simulink model "power_conversion_system"  (R2026a)
settings: Solver=VariableStepAuto  StopTime=100e-3  MaxStep=10e-6  MinStep=1e-9
values from neighbouring files (symbols this model uses):
  C_out1 = 100e-6    (= 0.0001)    [power_system_variables.m]
  L_boost1 = 1e-3    (= 0.001)    [power_system_variables.m]
  R_Load = 10    [power_system_variables.m]
  R_sense1 = 0.1    [power_system_variables.m]
  Vin = 12    [power_system_variables.m]
  Vout = 48    [power_system_variables.m]
undefined symbols (not defined in the file or in its folder): f_clk
settings Model: Creator=codykremer  LastModifiedBy=codykremer

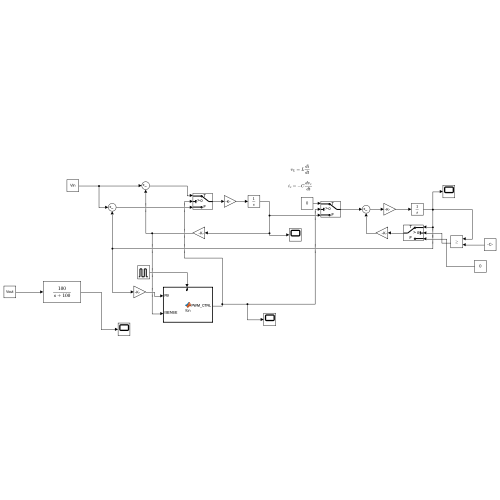
[thumbnail: Simulink's stored preview of the top-level diagram]
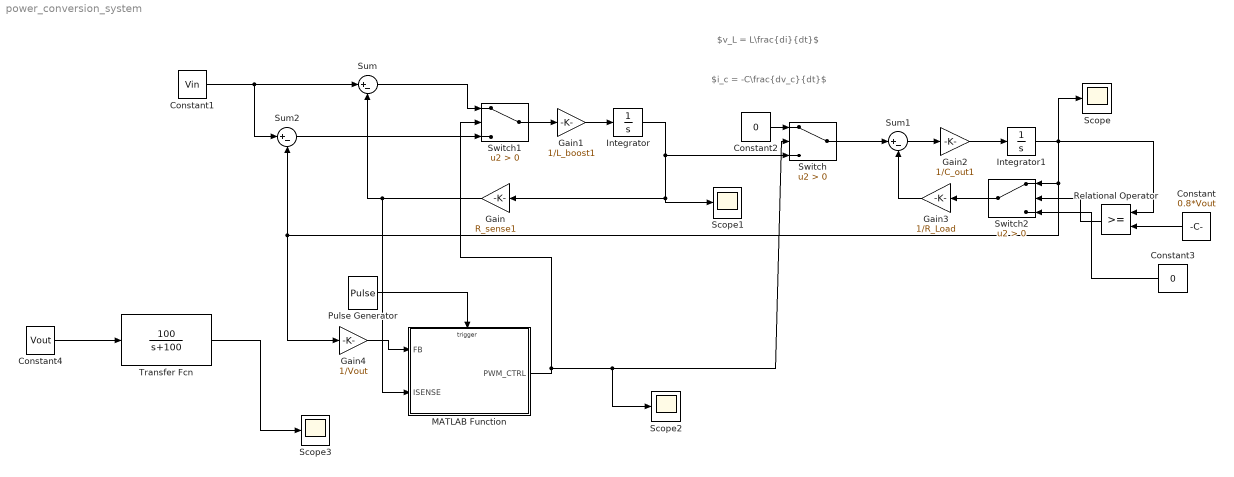
== system power_conversion_system ==
  note: $v_L = L\frac{di}{dt}$
  note: $i_c = -C\frac{dv_c}{dt}$
  Constant : Constant  Value=0.8*Vout  VectorParams1D=off
  Constant1 : Constant  Value=Vin
  Constant2 : Constant  Value=0
  Constant3 : Constant  Value=0  VectorParams1D=off
  Constant4 : Constant  Value=Vout
  Gain : Gain  Gain=R_sense1
  Gain1 : Gain  Gain=1/L_boost1
  Gain2 : Gain  Gain=1/C_out1
  Gain3 : Gain  Gain=1/R_Load
  Gain4 : Gain  Gain=1/Vout
  Integrator : Integrator
  Integrator1 : Integrator
  MATLAB Function : MATLAB Function  TreatAsAtomicUnit=on
  Pulse Generator : DiscretePulseGenerator  PulseType=Time based  Period=1/f_clk  PulseWidth=50
  Relational Operator : RelationalOperator  OutDataTypeStr=boolean  RndMeth=Simplest  InputSameDT=off
  Scope{,1..3} (4 alike) : Scope
      Scope settings: ActiveDisplayYMinimum=-3.0238183140973316  ActiveDisplayYMaximum=27.214364826875993
      Scope1 settings: ActiveDisplayYMinimum=-76.4299194528486  ActiveDisplayYMaximum=74.60389998830459
      Scope2 settings: ActiveDisplayYMinimum=-1  ActiveDisplayYMaximum=1  DataLoggingVariableName=ScopeData2
      Scope3 settings: ActiveDisplayYMinimum=-1  ActiveDisplayYMaximum=1  DataLoggingVariableName=ScopeData3
  Sum : Sum  Inputs=|+-
  Sum1 : Sum  Inputs=|+-
  Sum2 : Sum  Inputs=|+-
  Switch : Switch  Criteria=u2 > Threshold  SaturateOnIntegerOverflow=off  InputSameDT=off
  Switch1 : Switch  Criteria=u2 > Threshold  SaturateOnIntegerOverflow=off  InputSameDT=off
  Switch2 : Switch  Criteria=u2 > Threshold  SaturateOnIntegerOverflow=off  InputSameDT=off
  Transfer Fcn : TransferFcn  Numerator=[100]  Denominator=[1 100]
  wires:
  Sum1/1 -> Gain2/1
  Gain2/1 -> Integrator1/1
  Switch/1 -> Sum1/1
  Constant2/1 -> Switch/1
  Gain3/1 -> Sum1/2
  Constant1/1 -> Sum/1, Sum2/1
  Gain1/1 -> Integrator/1
  Sum/1 -> Switch1/1
  Integrator/1 -> Switch/3, Scope1/1, Gain/1
  Gain/1 -> Sum/2, MATLAB Function/2(ISENSE)
  Sum2/1 -> Switch1/3
  Switch1/1 -> Gain1/1
  Pulse Generator/1 -> MATLAB Function/Trigger
  MATLAB Function/1(PWM_CTRL) -> Scope2/1, Switch/2, Switch1/2
  Switch2/1 -> Gain3/1
  Constant/1 -> Relational Operator/2
  Relational Operator/1 -> Switch2/2
  Constant3/1 -> Switch2/3
  Integrator1/1 -> Relational Operator/1, Scope/1, Switch2/1, Gain4/1, Sum2/2
  Constant4/1 -> Transfer Fcn/1
  Gain4/1 -> MATLAB Function/1(FB)
  Transfer Fcn/1 -> Scope3/1

== matlab function power_conversion_system/MATLAB Function ==
  data: FB input; PWM_CTRL output; ISENSE input
  events: CLK input RISING_EDGE_EVENT
function PWM_CTRL  = fcn(FB, ISENSE)

    % COUNTER 
    persistent count; 
    if isempty(count) 
        count = 100;
    end
    count = mod(count + 1, 100);

    persistent DUTY;
    if isempty(DUTY)
        DUTY = 20;
    end
    
    if count < DUTY
        PWM_CTRL = 1;
    else
        PWM_CTRL = 0; 
    end

end
